simulink model "combined_models_v16"  (R2021a)
settings: Solver=VariableStepAuto  StartTime=0.0  StopTime=30  RelTol=1e-3
values from neighbouring files (symbols this model uses):
  r__s_st = r__s_stCG - r__t_tCG    [init_saildrone_dynamics_v5.m]    (also in moduleBasedModel_v7.m = cfg.r__s_st; systemVelocities.m = cfg.r__s_st)
  r__t_tAC = r__t_tCG    [init_saildrone_dynamics_v5.m]
  rho = 1025    [init_saildrone_dynamics_v5.m]    (also in moduleBasedModel_v7.m = cfg.rho; simplifiedModel_v8.m = cfg.rho)
  rho_air = 1.225    [init_saildrone_dynamics_v5.m]
undefined symbols (not defined in the file or in its folder): beta_V_w, cfg, delta_LOS, DiscIntNeverNeededParam, gamma_c, GWP, heading_controller_samplingtime, heading_rate_ref, K_b, K_d_heading, K_d_heading2, K_d_s, k_d_s, K_d_t, K_i_heading, K_i_heading2, K_i_s, k_i_s, K_i_t, K_p_heading, K_p_heading2, k_p_s, K_p_s, K_p_t, Ka_lin, keel, ObjectsPosition, omega_n_heading2, omega_n_s, q0, q_dot0, rudder, sail, sail_AOA_controller_samplingtime, sail_AOA_linearization_point, sail_AOA_saturation, sail_AOA_table, simulation_sampling_time, start_w_trans, tacking_minus, tacking_plus, tail, theta0, timeconstant_w, U_c, U_linearization_heading, U_w, U_w_step, v_current, v_wind, v_wind_unit, wn_ref_heading, wn_ref_t, xi0, zeta_ref_heading, zeta_ref_t
(part 3 of 3)

== matlab function combined_models_v16/Velocity logger3/MATLAB Function1 ==
  data: u input; U output; v input; beta_c output
function [U, beta_c] = speed(u,v)

U = sqrt(u^2 + v^2);
beta_c = atan2(v,u);

== matlab function combined_models_v16/sailsystem dynamics2/Sailsystem dynamics/MATLAB Function5 ==
  data: x input; x_dot output; v__n_rw input; delta_t input; r__s_stAC input; K_CL input; I_zz_ss input; beta_U_rw output
function [x_dot, beta_U_rw] = sailsystem_dynamics_LIN(x, v__n_rw, delta_t, r__s_stAC, K_CL, I_zz_ss)

[x_dot, beta_U_rw] = sailsystem_dynamics_LIN(x, v__n_rw, delta_t, r__s_stAC, K_CL, I_zz_ss);

== matlab function combined_models_v16/sailsystem dynamics2/Subsystem/MATLAB Function4 ==
  data: beta_U_r input; xi input; v__n_rw input; rho_air input; tau_sailsystem output; sail parameter; alpha_sail output
function [tau_sailsystem,alpha_sail] = sailForces(beta_U_r, xi,v__n_rw, rho_air ,sail)

% Relative Speed 
U_rw = sqrt(v__n_rw(1)^2 + v__n_rw(2)^2);
% % Parasitic drag of wing
% C_D_0 = sail.C_D_parasitic;

%% First order approximation of forces assuming U__rw change slowly so
% delta_U_rw is close to zero
% f__s_x = -(C_D_0*sail.S*rho_air*U_rw^2)/2;
% f__s_y = ((C_D_0*sail.S*rho_air)/2 - sail.K_C_L)*alpha_sail*U_rw^2;

%% approximation using small angles and a quadratic drag formulation
% C_d_quad = (sail.C_L_alpha^2)/(sail.AR*sail.e_OS*pi);
% % linar function of quadratic angle of attack
% f__s_x = -(U_rw^2)*(sail.S*rho_air*C_D_0/2 + (alpha_sail^2)*(sail.K_C_L + sail.S*rho_air*C_d_quad/2));
% % linear function of proportional AOA
% f__s_y = ((C_D_0*sail.S*rho_air)/2 - sail.K_C_L)*alpha_sail*U_rw^2;

% f__s_x = 0;

alpha_sail = ssa(beta_U_r - xi);
if norm(v__n_rw) < 0.0001
    alpha_sail = 0;
end

kappa_sail = sail.C_L_alpha/(pi*sail.e_OS*sail.AR);

% final expression assuming kappa is small
f__s_x = sail.K_C_L*((alpha_sail^2))*(1-kappa_sail)*(U_rw^2);
f__s_y = -sail.K_C_L*(alpha_sail)*U_rw^2;


tau_sailsystem = [f__s_x; f__s_y; 0; 0;0;0];

== matlab function combined_models_v16/Path Manager/Path Manager ==
  data: GWPs input; GWP output; local_path_complete input; GWP_index input; prev_GWP output; calulate_local_WPs output; GWP_index output
function [GWP, prev_GWP, calulate_local_WPs ,GWP_index] = fcn(GWPs, local_path_complete, GWP_index)

GWP = zeros(2,1);
prev_GWP = zeros(2,1);

calulate_local_WPs = 0;
if local_path_complete == 1
    GWP_index = GWP_index +1
    calulate_local_WPs = 1;
end

GWP(:,1) = GWPs(:,GWP_index+1);
prev_GWP(:,1) = GWPs(:,GWP_index);

== matlab function combined_models_v16/Heading PD control system1/SSA++2 ==
  data: heading_ref input; psi input; heading_ref_cor output; SSA_true input; last_error2 input; last_error2 output
function [heading_ref_cor, last_error2]  = SSARef(heading_ref, psi, SSA_true, last_error2)

% the SSA_ture = 0 means the SSA is off and input angle in -2pi to 2pi can
% be used for jibing


error_ssa = ssa(heading_ref - psi);
% error2 = mod(heading_ref - psi-2*pi, 4*pi)-2*pi;
if SSA_true == 1
    % the offset of using psi is removed as we add and subract the same
    % measurement
%     heading_ref_cor = error + psi;
%     last_psi = psi;
    heading_ref_cor = error_ssa + psi;
    last_error2 = heading_ref - psi; % store as reference for next jib
else
    error2 = mod(heading_ref - psi -  last_error2 -2*pi, 4*pi)-2*pi; % can only devaiate by 2 pi from previous regular SSA

    
%     error2 = mod(heading_ref - psi -2*pi, 4*pi)-2*pi;
    heading_ref_cor = error2 + (psi);
    
%     heading_ref_cor = error2 + psi;
%     heading_ref_cor = heading_ref;
%     heading_ref_cor =  error + psi - 2*pi*(2/pi)*atan(error)            %%mod(2*pi + error, 2*pi) + psi;
%     [M, I] = max([abs(heading_ref - psi),abs(2*pi+heading_ref - psi)]);
% %     heading_ref_cor = heading_ref -2*pi*sign(error); %psi+ 2*pi + error 
%     if I == 1
%         heading_ref_cor = heading_ref;
%     else
%         heading_ref_cor = mod(2*pi+heading_ref, 2*pi);
%     end
end
% if (heading_ref-psi) > pi
%     heading_ref_cor = heading_ref - 2*pi;
% elseif (heading_ref-psi) < pi
%     heading_ref_cor = heading_ref + 2*pi;
% else
%     heading_ref_cor = heading_ref;
% end

% y = ssa(error);

== matlab function combined_models_v16/Local path creator/MATLAB Function3 ==
  settings: updateMethod=DISCRETE  sampleTime=pathCreator_sampletime
  data: target_WP input; tacking_points_n output; prev_WP input; q input; chi input; beta_c input; U_c input; beta_w input; U_w input; tacking_minus input; tacking_plus input; circ_acceptance_R output; circ_acceptance_L output
function [tacking_points_n, circ_acceptance_R, circ_acceptance_L] = pathCreator2(target_WP, prev_WP, q, chi, beta_c, U_c, beta_w, U_w, tacking_minus, tacking_plus)
    [tacking_points_n, circ_acceptance_R, circ_acceptance_L] = pathCreator2(target_WP, prev_WP, q, chi, beta_c, U_c, beta_w, U_w, tacking_minus, tacking_plus);

== matlab function combined_models_v16/Heading PD control system1/MATLAB Function2 ==
  data: psi_d input; delta_r_d_bar output; psi_d_dot input; psi_d_ddot input; psi input; psi_dot input; U_rc_keel input; Kp input; Kd input; Ki input; int_e_alpha input; rudder parameter; cfg parameter; e_alpha output
function [delta_r_d_bar, e_alpha] = GSPID(psi_d, psi_d_dot, psi_d_ddot, psi, psi_dot, U_rc_keel, Kp, Kd, Ki, int_e_alpha, rudder, cfg)
% the GS PID part of the controller


U_rc_keel_star = max(U_rc_keel, 0.1); %7;max(U_rw_tail, 2);%15;%max(U_rw_tail, 2);

Ka = (cfg.r__b_brAC(1)^2)*rudder.K_C_L;
Kb = cfg.r__b_brAC(1)*rudder.K_C_L;


e_alpha = psi-psi_d;
e_alpha_dot = psi_dot-psi_d_dot; 

delta_r1 = -psi_dot*cfg.Nr/(rudder.K_C_L*cfg.r__b_brAC(1)*U_rc_keel_star);

M44 = cfg.M_SD(6,6);

% The controller (without the alpha_s_d feed forward)
% delta_r_d_bar = -( Ka*psi_d_dot/(Kb*U_rc_keel_star) + 2*Kd*e_alpha_dot/U_rc_keel_star + Kp*e_alpha + psi_d_ddot*M44/(Kb*U_rc_keel_star^2)+ U_rc_keel_star*Ki*int_e_alpha + delta_r1);
delta_r_d_bar = -( Ka*psi_d_dot/(Kb*U_rc_keel_star) + Kd*e_alpha_dot/U_rc_keel_star + Kp*e_alpha + psi_d_ddot*M44/(Kb*U_rc_keel_star^2)+ U_rc_keel_star*Ki*int_e_alpha + delta_r1);

%% antiwindup how will it be????


% shut down controller for small velocities, makes it a pure feed forward,
% need faiding here?
if U_rc_keel < 0.05
    delta_r_d_bar = 0;
end

% implement a set of alternative gain and faiding between?
% integrator and anti windup

% Faiding out the controller might not work with integrator?

== matlab function combined_models_v16/Subsystem/MATLAB Function ==
  data: eta input; nu input; eta_dot output
function eta_dot = J_THETA(eta,nu)
    % eta_dot = J_THETA(eta)*nu 2.53 FOSSEN

    phi = eta(4);
    theta = eta(5);
    psi = eta(6);
    
    J = eulerang(phi, theta, psi);
    
    eta_dot = J*nu;

== matlab function combined_models_v16/Heading PD control system1/Subsystem/heading reference model/MATLAB Function ==
  data: reference input; x_refmod_dot output; zeta_ref input; wn_ref input; x_refmod input
function x_refmod_dot  = refModelTail(reference, zeta_ref, wn_ref, x_refmod)

[x_refmod_dot] = referenceModelPA(reference, zeta_ref, wn_ref, x_refmod);

== matlab function combined_models_v16/Subsystem1/MATLAB Function ==
  data: target_WP input; chi_selected output; x__p_e output; y__p_e output; prev_WP input; q input; chi input; U_rc input; beta_c input; U_c input; beta_w input; U_w input; tacking_minus input; tacking_plus input; delta input; typeC input; prev_tacking input; tack_count input; tacking output; typeC output; prev_tacking output; tack_count output; prev_chi_selected input; prev_WP_update input; prev_WP_original input; prev_WP_update output; prev_WP_original output; ssa_on output; ssa_on input; jib_angle input; jib_angle output
function [chi_selected,x__p_e, y__p_e, tacking, typeC, prev_tacking, tack_count, prev_WP_update, prev_WP_original, ssa_on, jib_angle] = dynamicVMGPathExtendedClean(target_WP, prev_WP, q, chi, U_rc, beta_c, U_c, beta_w, U_w, tacking_minus, tacking_plus, delta ,typeC, prev_tacking, tack_count, prev_chi_selected, prev_WP_update, prev_WP_original, ssa_on, jib_angle)

[chi_selected,x__p_e, y__p_e, tacking, typeC, prev_tacking, tack_count, prev_WP_update, prev_WP_original, ssa_on, jib_angle] = dynamicVMGPathExtendedClean(target_WP, prev_WP, q, chi, U_rc, beta_c, U_c, beta_w, U_w, tacking_minus, tacking_plus, delta ,typeC, prev_tacking, tack_count, prev_chi_selected, prev_WP_update, prev_WP_original, ssa_on, jib_angle);

== matlab function combined_models_v16/Path Manager 2 for course selector/Path Manager ==
  data: q input; GWPs input; GWP output; GWP_index input; prev_GWP output; GWP_index output
function [GWP, prev_GWP ,GWP_index] = fcn(q, GWPs, GWP_index)

%% parameters
circ_accept = 20;

%% main
next_GWP_index = GWP_index + 1;

GWP = zeros(2,1);
prev_GWP = zeros(2,1);

% check circle of acceptance
next_GWP = GWPs(:,next_GWP_index);
position_error = [q(1); q(2)] - next_GWP;
error_norm = sqrt(position_error(1)^2 + position_error(2)^2);
   
if error_norm <= circ_accept
    GWP_index = GWP_index + 1   % set new wayspoints
    next_GWP_index = GWP_index+1;
end


GWP(:,1) = GWPs(:,next_GWP_index);
prev_GWP(:,1) = GWPs(:,GWP_index);

== matlab function combined_models_v16/Subsystem2/MATLAB Function ==
  settings: updateMethod=DISCRETE  sampleTime=5
  data: next_GWP output; prev_GWP output; q input; next_GWP input; prev_GWP input; x__p_e_prev input; y__p_e_prev input; object_locations_NED input; chi_commanded output; prev_GWP_update input; prev_GWP_original input; prev_GWP_update output; prev_GWP_original output; prev_path_state input; prev_path_state output; blocked_count input; blocked_count output
function [next_GWP, prev_GWP, chi_commanded, prev_GWP_update, prev_GWP_original, prev_path_state, blocked_count]  = colav(q, next_GWP, prev_GWP,  x__p_e_prev, y__p_e_prev, object_locations_NED, prev_GWP_update, prev_GWP_original, prev_path_state, blocked_count)


%% testparameters

x__n = q(1);
y__n = q(2);
theta = q(6);

% x__n = 000;
% y__n = 000;
% theta = -0*pi/4;
% next_GWP = [120; 0];
% prev_GWP = [0; 0];
% y__p_e_prev = -40;
% x__p_e_prev = 100;
gird_size = 1400;

%% Look for updates of WP
if prev_GWP_original == prev_GWP % Has the original changed?
    % no
    if isnan(prev_GWP_update(1)) 
        % prev_WP = prev_WP do nothing
    else                            % do we have a updated value?
        prev_GWP = prev_GWP_update;
    end
else
    % we have recived a new Global WP 
%     prev_WP = prev_WP; % us it
    prev_GWP_original = prev_GWP;  % update the new original
    prev_GWP_update = NaN(2,1);   % reset any updated value
end


%% map

% object_locations_NED = [300, 110; 
%                         1000, -500]

object_locations = [flip(object_locations_NED(:,1)'); flip(object_locations_NED(:,2)')];

map = binaryOccupancyMap(gird_size, gird_size, 1); %size and resolution in cells per meter
object_locations = object_locations + [gird_size/2, gird_size/2; gird_size/2, gird_size/2];
setOccupancy(map, object_locations, ones(2,1));
inflate(map, 20);

next_GWP_out = zeros(2,1);
prev_GWP_out = zeros(2,1);

[next_GWP, prev_GWP, chi_commanded, prev_path_state, blocked_count] = colavtesting5(x__n, y__n, theta, next_GWP, prev_GWP, map, x__p_e_prev, y__p_e_prev, gird_size, prev_path_state, blocked_count)


if prev_GWP ~= prev_GWP_original
    prev_GWP_update = prev_GWP
end

== matlab function combined_models_v16/Subsystem/Module based model ==
  data: q_ input; q_ddot output; q_dot input; v__b_c input; tau_sail_act input; tau_tail_act input; tau_keel input; tau_sail input; tau_tail input; tau_rudder input; cfg parameter; tau__b_rudder output
function [q_ddot, tau__b_rudder]= nonlinearSaildroneDynamics(q_, q_dot, v__b_c, tau_sail_act, tau_tail_act, tau_keel, tau_sail, tau_tail, tau_rudder, cfg)

    [q_ddot, tau__b_rudder] = moduleBasedModel_v7(q_, q_dot, v__b_c, tau_tail_act, tau_sail_act, tau_tail, tau_sail, tau_keel, tau_rudder, cfg);


% moduleBasedModel_v6 require system to have zero hight as it is a 2D
% representation without restoring forces

== matlab function combined_models_v16/Heading PD control system1/Subsystem/MATLAB Function ==
  data: integral_in input; integral_out output; e_delta_r input; delta_r_d_unsat input; delta_r_d output; h input; rudder_max input; rudder_stall input; M66 input; K_i_heading input
function [integral_out, delta_r_d] = SatAndAntiWindUP(integral_in, e_delta_r,delta_r_d_unsat, h, rudder_max, rudder_stall, M66, K_i_heading)


% function [tail_angle_d, integral_out] = SatAndAntiWindUP(tail_angle_d_unsat, e_alpha, U_rw_tail_star, U_rw_tail_star_prev, K_i_s, Kb, h, tail_angle_max, integral_in, cfg)
    % h = sampling time
    
    delta_r_d_stall = sign(delta_r_d_unsat)*rudder_stall;
    % is tail angle saturated?
    if K_i_heading == 0
        delta_r_d = delta_r_d_unsat;
        integral_out = 0;
    elseif abs(delta_r_d_unsat)> rudder_max
        % limit output
        delta_r_d = sign(delta_r_d_unsat)*rudder_max;
        
        % if tail angle is saturated, simply stop integrating
%         integral_out = integral_in;
        integral_out = integral_in - (1*h/K_i_heading)*(delta_r_d - delta_r_d_unsat);
        integral_out = integral_in - (1*h/K_i_heading)*(delta_r_d_stall - delta_r_d_unsat);
    elseif abs(delta_r_d_unsat) <= rudder_max  &&abs(delta_r_d_unsat)>= rudder_stall
        % ordinary output
        delta_r_d = delta_r_d_unsat;
%         delta_r_d_stall = sign(delta_r_d_unsat)*rudder_stall;
        
        % stop integrator at stall
%         integral_out = integral_in;
        integral_out = integral_in - (1*h/K_i_heading)*(delta_r_d_stall - delta_r_d_unsat);
    else
        delta_r_d = delta_r_d_unsat;
        % euler integration
        integral_out = integral_in + h*e_delta_r;
    end

== matlab function combined_models_v16/Heading PD control system1/Subsystem1/MATLAB Function1 ==
  data: u input; U_linearization_heading input; y output; rudder parameter; cfg parameter
function y  = fcn(u,U_linearization_heading,rudder, cfg)

y = u/(-rudder.K_C_L*(cfg.r__b_brAC(1))*U_linearization_heading);

% rudderk = rudder.K_C_L;
% r__b = cfg.r__b_brAC(1);
% U_linearization_heading = U_linearization_heading;


% rudderk, r__b, U_linearization_heading

== matlab function combined_models_v16/Heading PD control system1/Subsystem1/SSA++1 ==
  data: heading_ref input; psi input; error input; y output
function y  = fcn(heading_ref, psi, error)

if abs(heading_ref-psi) > pi
    y = -error;
%     y_dot = -error_dot;
else
    y = ssa(error);
%     y_dot = error;
end

% y = ssa(error);

== matlab function combined_models_v16/Heading PD control system1/Subsystem1/SSA1 ==
  data: error input; y output
function y = fcn(error)

% y = error;
y = ssa(error);

== matlab function combined_models_v16/Heading PD control system1/Gain scheduler1/MATLAB Function ==
  data: U_rc input; omega_n_s input; wn_ref_sAOA output; zeta_ref_sAOA output; cfg parameter
function [wn_ref_sAOA, zeta_ref_sAOA] = RMS(U_rc, omega_n_s, cfg)
% reference model schedular

% Change reference model with velocity to adjust reference model to the
% sailsystems changing bandwidth 

               
omega_n_s = U_rc*omega_n_s;%sqrt((-Kb*(U_rw_sail^2)*(1+Kp))/cfg.I__PP_sailsystem(3,3));
%% Sail AOA reference model

% adjust reference model with respect to current system dynnamics, allow
% 10% margin for tracking controll
wn_ref_sAOA = omega_n_s*0.5;
wn_ref_sAOA_max = 2*pi/10;%2*pi/15;

wn_ref_sAOA = min(wn_ref_sAOA, wn_ref_sAOA_max);
zeta_ref_sAOA = 1;

== matlab function combined_models_v16/Heading PD control system1/heading reference model1/MATLAB Function ==
  data: reference input; x_refmod_dot output; zeta_ref input; wn_ref input; x_refmod input
function x_refmod_dot  = refModelTail(reference, zeta_ref, wn_ref, x_refmod)

[x_refmod_dot] = referenceModelPA(reference, zeta_ref, wn_ref, x_refmod);

== matlab function combined_models_v16/VMG ==
  data: target_WP input; VMG output; prev_WP input; chi input; q_dot input
function VMG = fcn(target_WP, prev_WP, chi, q_dot)

magnitude = sqrt(q_dot(1)^2 + q_dot(2)^2);
chi_target_d = atan2(target_WP(2)-prev_WP(2), target_WP(1)-prev_WP(1));

VMG = magnitude*cos(chi_target_d- chi);

== matlab function combined_models_v16/Subsystem/v_wind/MATLAB Function1 ==
  data: a input; y output; b input
function y = fcn(a,b)

y = a.*b;

== matlab function combined_models_v16/v_wind/MATLAB Function3 ==
  data: a input; y output; b input
function y = fcn(a,b)

y = a.*b;

== matlab function combined_models_v16/Subsystem/Velocity logger/U ==
  data: u input; U output; v input; beta_c output
function [U, beta_c] = speed(u,v)

U = sqrt(u^2 + v^2);
beta_c = atan2(v,u);

== matlab function combined_models_v16/Subsystem/MATLAB Function3 ==
  data: q_ input; nu_keelAC output; q_dot input; q_4_dot input; cfg parameter; nu_sailAC output; nu_tailAC output; nu_rudderAC output; v__n_sailAC output
function [nu_keelAC, nu_sailAC, nu_tailAC, nu_rudderAC, v__n_sailAC] = systemVelocities(q_, q_dot, q_4_dot, cfg)

 [nu_keelAC, nu_sailAC, nu_tailAC, nu_rudderAC, v__n_sailAC] = systemVelocities(q_, q_dot, q_4_dot, cfg);

== matlab function combined_models_v16/tail angle control system/Tail angle controller/MATLAB Function ==
  data: alpha_t input; U_rw_tail input; tau_windM output; cfg parameter; tail parameter
function tau_windM = windMoment(alpha_t,U_rw_tail, cfg, tail)

% Distance from actuator axis to AC of tail:
l_t_AC = abs(cfg.r__t_tAC(1));

tau_windM = tail.K_C_L*(U_rw_tail^2)*sin(alpha_t)*l_t_AC;
